simulink model "linear_Kalman_heli"  (R2017a)
settings: Solver=ode4  StartTime=0.0  StopTime=inf  FixedStep=0.1  RelTol=1e-3
InitFcn:
  | initialize_simulation
libraries: realtime_pacer_lib x1
settings Model: Creator=rosha  LastModifiedBy=rosha

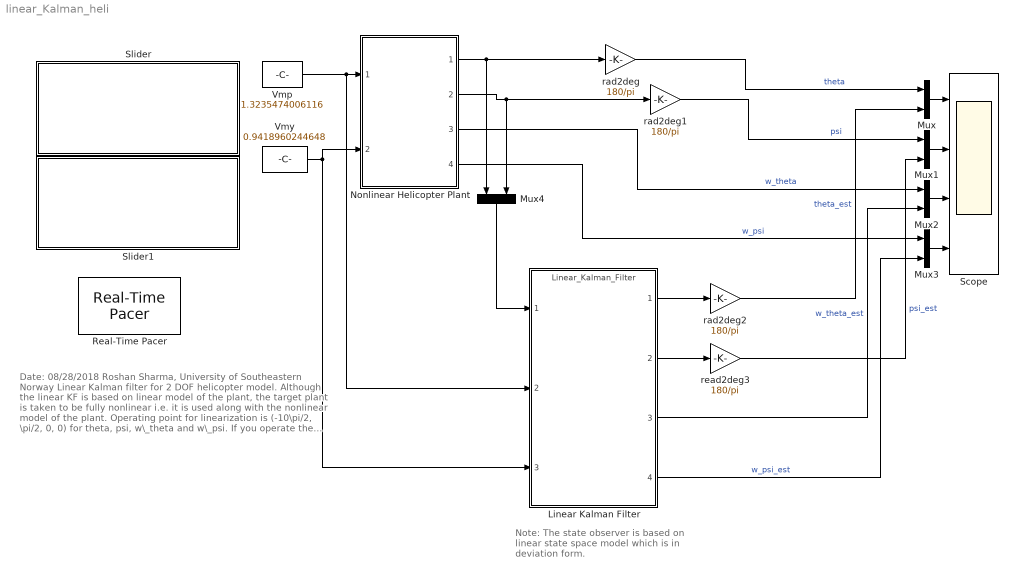
== system linear_Kalman_heli ==
  note: Date: 08/28/2018
      | Roshan Sharma, University of Southeastern Norway
      |
      | Linear Kalman filter for 2 DOF helicopter model.
      | Although the linear KF is based on linear model of the plant,
      | the target plant is taken to be fully nonlinear i.e. it is used along
      | with the nonlinear model of the plant.
      |
      | Operating point for linearization is (-10\pi/2, \pi/2, 0, 0) for theta,
      | psi, w\_theta and w\_psi.
      |
      | If you operate the helicopter far away from the operating point,
      | the linear KF will produce offset, which is very normal.
      |
      | UKF performs better than the linear KF under such conditions.
  note: Note: The state observer is based on
      | linear state space model which is
      | in deviation form.
  Linear Kalman Filter : ModelReference  ModelNameDialog=Linear_Kalman_Filter  ModelReferenceVersion=1.50  CopyOfModelProtected=on
  Mux{,1..4} (5 alike) : Mux  Inputs=2
  Nonlinear Helicopter Plant : ModelReference  ModelNameDialog=Nonlinear_Helicopter_Plant  ModelReferenceVersion=1.53  CopyOfModelProtected=on
  Real-Time Pacer : realtime_pacer_lib/Real-Time Pacer  simTimePerRealTime=1
  Scope : Scope  NumInputPorts=4
  Slider : Subsystem  DialogController=hmiCreateDDGDialog  IsWebBlock=on  mask(MWDashboardBlock){webBlockId=65708a0b-0db9-4818-99ef-91d910a647f9, webBlockType=slider, ShowInLibBrowser=on, ShowInitialText=on, HMISrcModelName=linear_observer_heli}
      mask prompts: webBlockId "WebBlock Id"; webBlockType "WebBlock Type"; HMISrcModelName "Source Model"
      mask help: SimulinkHMI:dialogs:SliderDialogDesc
      mask Help: helpview([docroot '/mapfiles/simulink.map'], 'hmi_slider')
      mask Display:
      | if strcmp(get_param(bdroot(gcb),'BlockDiagramType'), 'library')
      |     image([(matlabroot) '/toolbox/simulink/hmi/icons/Slider.png']);
      | end
  Slider1 : Subsystem  DialogController=hmiCreateDDGDialog  IsWebBlock=on  mask(MWDashboardBlock){webBlockId=0ca4703d-b5a7-41b4-b347-6eb94f80e79f, webBlockType=slider, ShowInLibBrowser=on, ShowInitialText=on, HMISrcModelName=linear_observer_heli}
      mask prompts: webBlockId "WebBlock Id"; webBlockType "WebBlock Type"; HMISrcModelName "Source Model"
      mask help: SimulinkHMI:dialogs:SliderDialogDesc
      mask Help: helpview([docroot '/mapfiles/simulink.map'], 'hmi_slider')
      mask Display:
      | if strcmp(get_param(bdroot(gcb),'BlockDiagramType'), 'library')
      |     image([(matlabroot) '/toolbox/simulink/hmi/icons/Slider.png']);
      | end
  Vmp : Constant  Value=1.3235474006116
  Vmy : Constant  Value=0.9418960244648
  rad2deg : Gain  Gain=180/pi
  rad2deg1 : Gain  Gain=180/pi
  rad2deg2 : Gain  Gain=180/pi
  read2deg3 : Gain  Gain=180/pi
  wires:
  Mux/1 -> Scope/1
  Nonlinear Helicopter Plant/1 -> Mux4/1, rad2deg/1
  rad2deg/1 -> Mux/1  "theta"
  Nonlinear Helicopter Plant/2 -> rad2deg1/1, Mux4/2
  Nonlinear Helicopter Plant/3 -> Mux2/1  "w_theta"
  rad2deg2/1 -> Mux/2  "theta_est"
  Mux1/1 -> Scope/2
  rad2deg1/1 -> Mux1/1  "psi"
  read2deg3/1 -> Mux1/2  "psi_est"
  Mux2/1 -> Scope/3
  Mux3/1 -> Scope/4
  Nonlinear Helicopter Plant/4 -> Mux3/1  "w_psi"
  Vmp/1 -> Linear Kalman Filter/2, Nonlinear Helicopter Plant/1
  Vmy/1 -> Linear Kalman Filter/3, Nonlinear Helicopter Plant/2
  Mux4/1 -> Linear Kalman Filter/1
  Linear Kalman Filter/3 -> Mux2/2  "w_theta_est"
  Linear Kalman Filter/4 -> Mux3/2  "w_psi_est"
  Linear Kalman Filter/1 -> rad2deg2/1
  Linear Kalman Filter/2 -> read2deg3/1

== system linear_Kalman_heli/Slider ==

== system linear_Kalman_heli/Slider1 ==
